simulink model "complete_open_loop_model_1_4"  (R2025b)
settings: Solver=VariableStepAuto  StartTime=0.0  StopTime=200  RelTol=1e-3
undefined symbols (not defined in the file or in its folder): alpha, Den, eta_0, Jr, Js, Num, omega, sigma_m_square, taue, taum, Tc_max, Torque_disturbance, wr_max, xi
libraries: SignalEditorBlockLib x1
settings Model: Creator=flori  LastModifiedBy=flori

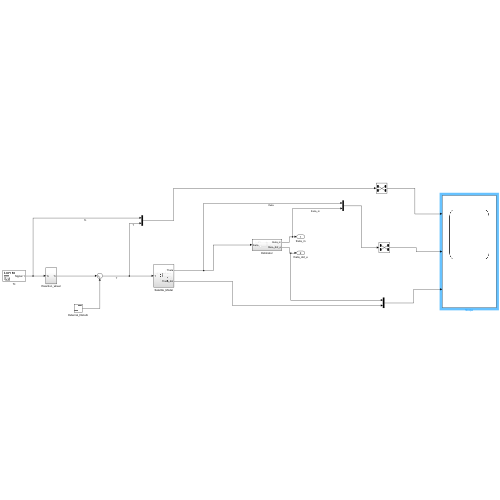
[thumbnail: Simulink's stored preview of the top-level diagram]
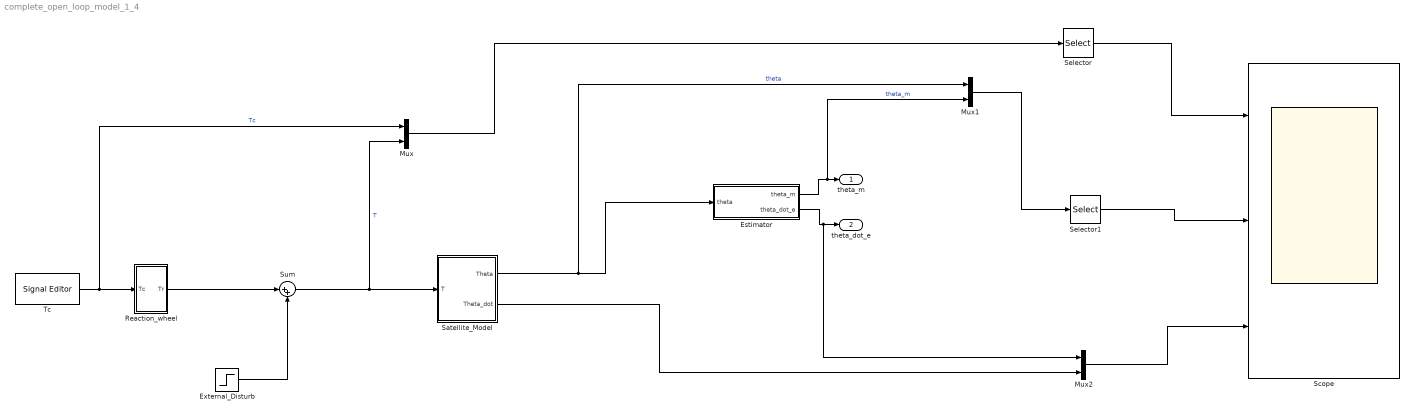
== system complete_open_loop_model_1_4 ==
  Estimator : Subsystem
  External_Disturb : Step  Time=100  After=Torque_disturbance  SampleTime=0
  Mux : Mux  Inputs=2
  Mux1 : Mux  Inputs=2
  Mux2 : Mux  Inputs=2
  Reaction_wheel : Subsystem
  Satellite_Model : Subsystem
  Scope : Scope  NumInputPorts=3
      settings: ActiveDisplayString=3  ActiveDisplayYMinimum=-0.033587721309730541  ActiveDisplayYMaximum=0.05885932778504669
  Selector : Selector  InputPortWidth=2  IndexOptions=Index vector (dialog)  Indices=[2 1]  OutputSizes=1
  Selector1 : Selector  InputPortWidth=2  IndexOptions=Index vector (dialog)  Indices=[2 1]  OutputSizes=1
  Sum : Sum  Inputs=|++
  Tc : SignalEditorBlockLib/Signal Editor  FileName=square signal.mat  ActiveScenario=Scenario  ActiveSignal=Signal 1  IsBus=off  OutputBusObjectStr=Bus: BusObject  SampleTime=0  ZeroCross=off  OutputAfterFinalValue=Setting to zero  Unit=inherit  PreserveSignalName=on  ApplySigPropsToAllScenarios=on  ApplySigPropsToAllSignals=off  SignalPropertySource=Dialog parameters
  theta_m : Outport
  theta_dot_e : Outport  Port=2
  wires:
  Estimator/1(theta_m) -> Mux1/2, theta_m/1  "theta_m"
  Estimator/2(theta_dot_e) -> Mux2/1, theta_dot_e/1
  Reaction_wheel/1(Tr) -> Sum/1
  Sum/1 -> Mux/2, Satellite_Model/1(T)  "T"
  Satellite_Model/1(Theta) -> Mux1/1, Estimator/1(theta)  "theta"
  Tc/1 -> Mux/1, Reaction_wheel/1(Tc)  "Tc"
  External_Disturb/1 -> Sum/2
  Mux/1 -> Selector/1
  Mux1/1 -> Selector1/1
  Satellite_Model/2(Theta_dot) -> Mux2/2
  Mux2/1 -> Scope/3
  Selector/1 -> Scope/1
  Selector1/1 -> Scope/2

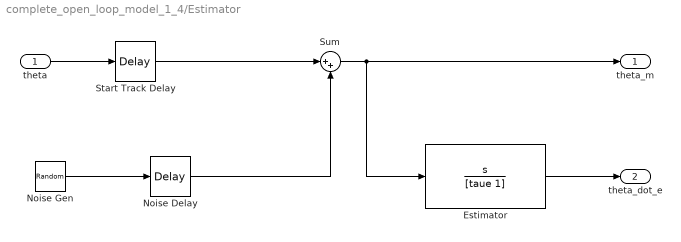
== system complete_open_loop_model_1_4/Estimator ==
  theta : Inport
  Estimator : TransferFcn  Numerator=[1 0]  Denominator=[taue 1]
  Noise Delay : TransportDelay  DelayTime=160
  Noise Gen : RandomNumber  Variance=sigma_m_square  SampleTime=0.01
  Start Track Delay : TransportDelay  DelayTime=taum
  Sum : Sum  Inputs=|++
  theta_m : Outport
  theta_dot_e : Outport  Port=2
  wires:
  Start Track Delay/1 -> Sum/1
  Sum/1 -> theta_m/1, Estimator/1
  theta/1 -> Start Track Delay/1
  Estimator/1 -> theta_dot_e/1
  Noise Gen/1 -> Noise Delay/1
  Noise Delay/1 -> Sum/2

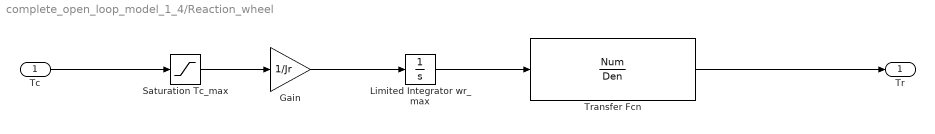
== system complete_open_loop_model_1_4/Reaction_wheel ==
  Tc : Inport
  Gain : Gain  Gain=1/Jr
  Limited Integrator wr_max : Integrator  LimitOutput=on  UpperSaturationLimit=wr_max  LowerSaturationLimit=-wr_max
  Saturation Tc_max : Saturate  UpperLimit=Tc_max  LowerLimit=-Tc_max
  Transfer Fcn : TransferFcn  Numerator=Num  Denominator=Den
  Tr : Outport
  wires:
  Saturation Tc_max/1 -> Gain/1
  Gain/1 -> Limited Integrator wr_max/1
  Limited Integrator wr_max/1 -> Transfer Fcn/1
  Transfer Fcn/1 -> Tr/1
  Tc/1 -> Saturation Tc_max/1

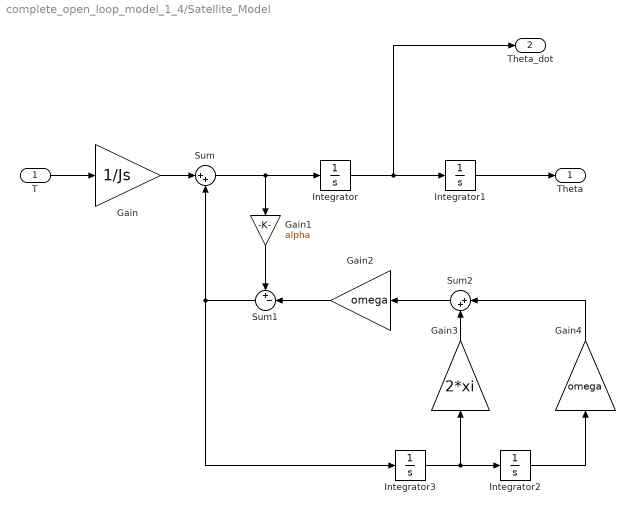
== system complete_open_loop_model_1_4/Satellite_Model ==
  T : Inport
  Gain : Gain  Gain=1/Js
  Gain1 : Gain  Gain=alpha
  Gain2 : Gain  Gain=omega
  Gain3 : Gain  Gain=2*xi
  Gain4 : Gain  Gain=omega
  Integrator : Integrator
  Integrator1 : Integrator
  Integrator2 : Integrator  InitialCondition=eta_0
  Integrator3 : Integrator
  Sum : Sum  Inputs=|++
  Sum1 : Sum  Inputs=+-|
  Sum2 : Sum  Inputs=|++
  Theta : Outport
  Theta_dot : Outport  Port=2
  wires:
  Integrator/1 -> Theta_dot/1, Integrator1/1
  Gain4/1 -> Sum2/1
  Sum/1 -> Gain1/1, Integrator/1
  Gain2/1 -> Sum1/2
  Sum1/1 -> Integrator3/1, Sum/2
  Gain1/1 -> Sum1/1
  Gain3/1 -> Sum2/2
  Integrator3/1 -> Integrator2/1, Gain3/1
  Sum2/1 -> Gain2/1
  T/1 -> Gain/1
  Integrator1/1 -> Theta/1
  Gain/1 -> Sum/1
  Integrator2/1 -> Gain4/1
